simulink model "battery_charging_new"  (R2023a)
settings: Solver=ode23tb  StartTime=0.0  StopTime=350  RelTol=1e-3
undefined symbols (not defined in the file): Ion, Lithium
libraries: spsSeriesRLCBranchLib x3, spsCurrentMeasurementLib x2, spsDiodeLib x2, spsVoltageMeasurementLib x2, spsBatteryLib x1, spsMosfetLib x1, spsPVArrayLib x1, spsPWMGeneratorDCDCLib x1, spspowerguiLib x1
settings Model: Creator=mluser  LastModifiedBy=mluser
settings SolverCC: ZeroCrossAlgorithm=Adaptive
settings DebuggingCC: IgnoredZcDiagnostic=none

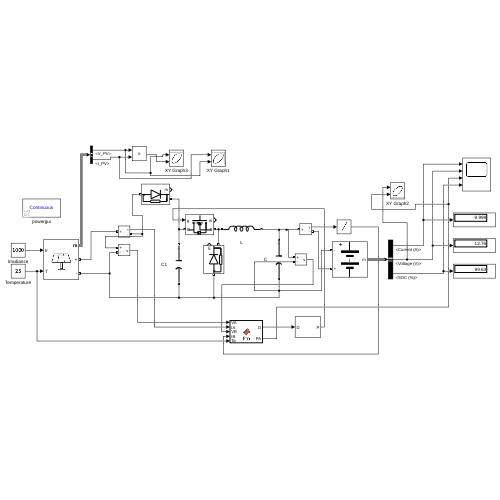
[thumbnail: Simulink's stored preview of the top-level diagram]
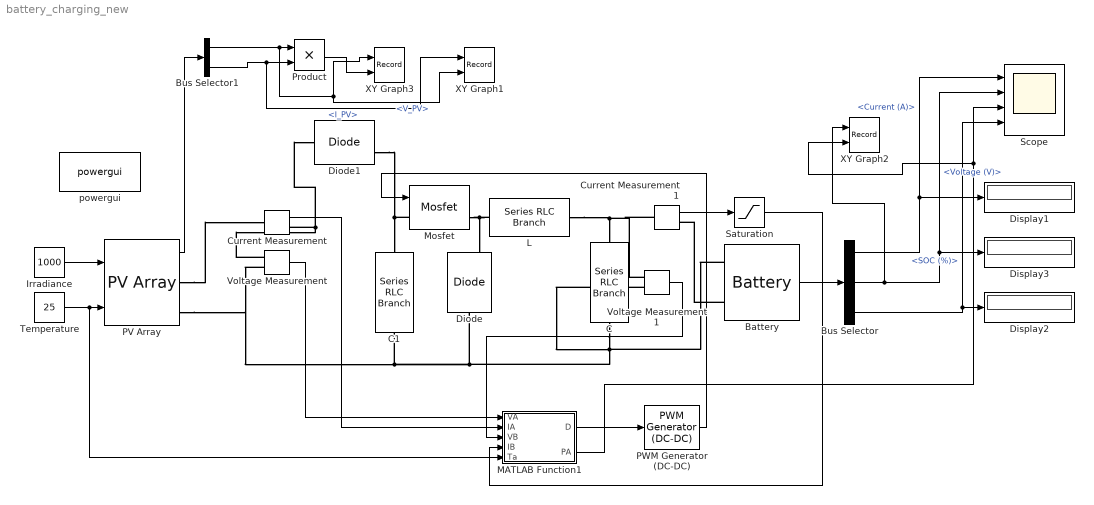
== system battery_charging_new ==
  Battery : spsBatteryLib/Battery  BatType=Lithium-Ion  ShowTempParam=off  ThermalPreset=no  ShowAgeParam=off  NomV=12  NomQ=50  SOC=99.6  Batt_Tr=30  PresetModel=off  MaxQ=50  MinV=9  FullV=14.4  Dis_rate=10  R=0.024  Normal_OP=25  expZone="[12.2171    0.166667]"  current=[6.5 13 32.5]  Units=Time  Tci=20  NomT=20  T2=-30  MaxQ2=4.8  FullV2=7.1  Normal_OP2=5.655  expZone2="[6.58           1]"  Rca=0.6  ti=2000  Dp=0  Neq0=0  Tsim=1e6  Ta1=25  Qeol=5.4*0.9  Reol=0.013333*1.2  Char_age=[2.3478, 3]  Dis_age=[2.3478, 10]  N1=1500  N2=10500  N3=1000  N4=1400  Ta2=45  N5=950
  Bus Selector : BusSelector  OutputSignals=Current (A),Voltage (V),SOC (%)
  Bus Selector1 : BusSelector  OutputSignals=V_PV,I_PV
  C : spsSeriesRLCBranchLib/Series RLC Branch  LConnTagsString=__new0  RConnTagsString=__new0  BranchType=C  Resistance=1  Inductance=1e-3  SetiL0=off  InitialCurrent=0  Capacitance=1000e-6  Setx0=off  InitialVoltage=0  Measurements=None
  C1 : spsSeriesRLCBranchLib/Series RLC Branch  LConnTagsString=__new0  RConnTagsString=__new0  BranchType=C  Resistance=1  Inductance=1e-3  SetiL0=off  InitialCurrent=0  Capacitance=1000e-6  Setx0=off  InitialVoltage=0  Measurements=None
  Current Measurement : spsCurrentMeasurementLib/Current Measurement  PhasorSimulation=off  OutputType=Complex  PSBequivalent=0
  Current Measurement1 : spsCurrentMeasurementLib/Current Measurement  PhasorSimulation=off  OutputType=Complex  PSBequivalent=0
  Diode : spsDiodeLib/Diode  Ron=0.001  Lon=0  Vf=0.8  IC=0  UseSnubber=0  Rs=500  Cs=250e-9  Measurements=on
  Diode1 : spsDiodeLib/Diode  Ron=0.001  Lon=0  Vf=0.8  IC=0  UseSnubber=0  Rs=500  Cs=250e-9  Measurements=on
  Display1 : Display
  Display2 : Display
  Display3 : Display
  Irradiance : Constant  Value=1000
  L : spsSeriesRLCBranchLib/Series RLC Branch  LConnTagsString=__new0  RConnTagsString=__new0  BranchType=L  Resistance=1  Inductance=10e-3  SetiL0=off  InitialCurrent=0  Capacitance=1e-6  Setx0=off  InitialVoltage=0  Measurements=None
  MATLAB Function1 : MATLAB Function  TreatAsAtomicUnit=on
  Mosfet : spsMosfetLib/Mosfet  Ron=0.1  Lon=0  Rd=0.01  Vfd=0  IC=0  Rs=1e5  Cs=inf  Measurements=on
  PV Array : spsPVArrayLib/PV Array  Npar=1  Nser=1  PlotType=array @ 1000 W/m2 & specified temperatures  S_vec="[ 1000  500  100 ]"  Temp_C_vec="[ 45 25  ]"  ModuleName=Canadian Solar Inc. CS6P-240MX  PlotWhenSelected=off  Pm=240.09  Ncell=60  Voc=37.3  Isc=8.46  Vm=30.2  Im=7.95  beta_Voc_pc=-0.35  alpha_Isc_pc=0.04  beta_Voc=-0.13055  alpha_Isc=0.003384  IL=8.4716  I0=1.9544e-10  nI=0.98841  Rsh=369.5316  Rs=0.32617  RobustModel=off  RobustCellTemperature=313.3991  BAL=on  Tc=1e-6  Tfilter=5e-5
  PWM Generator (DC-DC) : spsPWMGeneratorDCDCLib/PWM Generator (DC-DC)  Fsw=40000  Ts=0
  Product : Product
  Saturation : Saturate  UpperLimit=50  LowerLimit=0
  Scope : Scope  NumInputPorts=4
  Temperature : Constant  Value=25
  Voltage Measurement : spsVoltageMeasurementLib/Voltage Measurement  PhasorSimulation=off  OutputType=Complex  PSBequivalent=0
  Voltage Measurement1 : spsVoltageMeasurementLib/Voltage Measurement  PhasorSimulation=off  OutputType=Complex  PSBequivalent=0
  XY Graph1 : Record  FileSettingsInternal="{\"entries\":[{\"content\":{\"excelSettings\":{\"content\":{},\"type\":\"Streamout.ExcelSettings\"}},\"type\":\"Streamout.FileSettingStorage\",\"uuid\":\"\"}],\"packageUris\":[\"http:\\/\\/schema.mathworks.com\\/mf0\\/streamout_blocks\\/R2020a\"],\"version\":\"1.0\"}"  Layout=[1 1]  SignalsInternal="{\"entries\":[{\"content\":{\"signals\":[{\"content\":{\"blockPath\":[],\"dimensions\":[1],\"domain\":\"\",\"lineColor\":\"#a2142f\",\"plots\":[1],\"port\":1,\"sid\":[\"\"],\"signalID\":1211,\"signalName\":\"<I_PV>\"},\"type\":\"RecordBlkView.Signal\",\"uuid\":\"\"},{\"content\":{\"blockPath\":[],\"dimensions\":[1],\"domain\":\"\",\"lineColor\":\"#139fff\",\"plots\":[1],\"port\":2,\"sid\":[\"\"],\"signalID\":1215,\"signalName\":\"<V_PV>\"},\"type\":\"RecordBlkView.Signal\",\"uuid\":\"\"}]},\"type\":\"RecordBlkView.InputSignals\",\"uuid\":\"\"}],\"packageUris\":[\"http:\\/\\/schema.mathworks.com\\/mf0\\/streamout_blocks\\/R2020a\"],\"version\":\"1.0\"}"  VisualizationBindings="{\"xyplotplugin\":{\"info\":[{\"series\":[{\"bindingParametersList\":[{\"parameter\":\"X-Axis\",\"signalID\":1211,\"signalName\":\"<I_PV>\"},{\"parameter\":\"Y-Axis\",\"signalID\":1215,\"signalName\":\"<V_PV>\"}],\"seriesID\":56904}],\"subplotID\":1}]}}"  CompatibilityTag=XY  st=-1
  XY Graph2 : Record  FileSettingsInternal="{\"entries\":[{\"content\":{\"excelSettings\":{\"content\":{},\"type\":\"Streamout.ExcelSettings\"}},\"type\":\"Streamout.FileSettingStorage\",\"uuid\":\"\"}],\"packageUris\":[\"http:\\/\\/schema.mathworks.com\\/mf0\\/streamout_blocks\\/R2020a\"],\"version\":\"1.0\"}"  Layout=[1 1]  SignalsInternal="{\"entries\":[{\"content\":{\"signals\":[{\"content\":{\"blockPath\":[],\"dimensions\":[1],\"domain\":\"\",\"lineColor\":\"#a2142f\",\"plots\":[1],\"port\":1,\"sid\":[\"\"],\"signalID\":1219,\"signalName\":\"<Voltage (V)>\"},\"type\":\"RecordBlkView.Signal\",\"uuid\":\"\"},{\"content\":{\"blockPath\":[],\"dimensions\":[1],\"domain\":\"\",\"lineColor\":\"#139fff\",\"plots\":[1],\"port\":2,\"sid\":[\"\"],\"signalID\":1223,\"signalName\":\"MATLAB Function1:2\"},\"type\":\"RecordBlkView.Signal\",\"uuid\":\"\"}]},\"type\":\"RecordBlkView.InputSignals\",\"uuid\":\"\"}],\"packageUris\":[\"http:\\/\\/schema.mathworks.com\\/mf0\\/streamout_blocks\\/R2020a\"],\"version\":\"1.0\"}"  VisualizationBindings="{\"xyplotplugin\":{\"info\":[{\"series\":[{\"bindingParametersList\":[{\"parameter\":\"X-Axis\",\"signalID\":1219,\"signalName\":\"<Voltage (V)>\"},{\"parameter\":\"Y-Axis\",\"signalID\":1223,\"signalName\":\"MATLAB Function1:2\"}],\"seriesID\":36722}],\"subplotID\":1}]}}"  CompatibilityTag=XY  st=-1
  XY Graph3 : Record  FileSettingsInternal="{\"entries\":[{\"content\":{\"excelSettings\":{\"content\":{},\"type\":\"Streamout.ExcelSettings\"}},\"type\":\"Streamout.FileSettingStorage\",\"uuid\":\"\"}],\"packageUris\":[\"http:\\/\\/schema.mathworks.com\\/mf0\\/streamout_blocks\\/R2020a\"],\"version\":\"1.0\"}"  Layout=[1 1]  SignalsInternal="{\"entries\":[{\"content\":{\"signals\":[{\"content\":{\"blockPath\":[],\"dimensions\":[1],\"domain\":\"\",\"lineColor\":\"#a2142f\",\"plots\":[1],\"port\":1,\"sid\":[\"\"],\"signalID\":1227,\"signalName\":\"<V_PV>\"},\"type\":\"RecordBlkView.Signal\",\"uuid\":\"\"},{\"content\":{\"blockPath\":[],\"dimensions\":[1],\"domain\":\"\",\"lineColor\":\"#139fff\",\"plots\":[1],\"port\":2,\"sid\":[\"\"],\"signalID\":1231,\"signalName\":\"Product\"},\"type\":\"RecordBlkView.Signal\",\"uuid\":\"\"}]},\"type\":\"RecordBlkView.InputSignals\",\"uuid\":\"\"}],\"packageUris\":[\"http:\\/\\/schema.mathworks.com\\/mf0\\/streamout_blocks\\/R2020a\"],\"version\":\"1.0\"}"  VisualizationBindings="{\"xyplotplugin\":{\"info\":[{\"series\":[{\"bindingParametersList\":[{\"parameter\":\"X-Axis\",\"signalID\":1227,\"signalName\":\"<V_PV>\"},{\"parameter\":\"Y-Axis\",\"signalID\":1231,\"signalName\":\"Product\"}],\"seriesID\":53361}],\"subplotID\":1}]}}"  CompatibilityTag=XY  st=-1
  powergui : spspowerguiLib/powergui  Priority=1  SimulationMode=Continuous  SampleTime=1e-6  frequency=60  Iterations=50  frequencyindice=0  Pbase=100e6  ErrMax=1e-4  UnitsV=kV  UnitsW=MW  buscounter=0  FunctionMessages=off  echomessages=off  EnableUseOfTLC=off  CurrentSourceSwitches=off  DisableSnubberDevices=off  DisableRonSwitches=off  DisableVfSwitches=off  DisplayEquations=off  AutomaticDiscreteSolvers=off  SolverType=Tustin/Backward Euler (TBE)  Interpol=off  ExternalGateDelay=off  methode=off  Ts=100  x0status=blocks  SPID=on  SwTol=0  HookPort=off  NonlinearTolerance=1e-4  nMaxIteration=100  ContinueOnMaxIteration=off  RestoreLinks=warning  ResistiveCurrentMeasurement=off  Frange=[0:2:500]  Ylog=off  Xlog=on  ShowGrid=off  save=off  variable=ZData  structure=0  ZoomFFT=off  StartTime=0.0  cycles=1  DisplayStyle=1  fundamental=60  FreqAxis=off  MaxFrequency=1000  frequencyindicesteady=1  RmsSteady=1  display=off
  wires:
  Battery/1 -> Bus Selector/1
  Bus Selector/2 -> XY Graph2/1, Scope/2, Display3/1  "<Voltage (V)>"
  Bus Selector/3 -> Display2/1, Scope/4  "<SOC (%)>"
  Temperature/1 -> MATLAB Function1/5(Ta), PV Array/2
  Irradiance/1 -> PV Array/1
  Bus Selector/1 -> Scope/1, Display1/1  "<Current (A)>"
  Current Measurement/1 -> MATLAB Function1/2(IA)
  Voltage Measurement1/1 -> MATLAB Function1/3(VB)
  Voltage Measurement/1 -> MATLAB Function1/1(VA)
  MATLAB Function1/1(D) -> PWM Generator (DC-DC)/1
  PWM Generator (DC-DC)/1 -> Mosfet/1
  MATLAB Function1/2(PA) -> XY Graph2/2, Scope/3
  Current Measurement1/1 -> Saturation/1
  Saturation/1 -> MATLAB Function1/4(IB)
  PV Array/1 -> Bus Selector1/1
  Bus Selector1/1 -> XY Graph1/2, XY Graph3/1, Product/1  "<V_PV>"
  Bus Selector1/2 -> XY Graph1/1, Product/2  "<I_PV>"
  Product/1 -> XY Graph3/2
  connections:
  Mosfet/RConn1 -- L/LConn1 -- Diode/RConn1
  Battery/LConn2 -- Voltage Measurement1/LConn2 -- Voltage Measurement/LConn2 -- PV Array/RConn2 -- C1/RConn1 -- Diode/LConn1 -- C/RConn1
  L/RConn1 -- Current Measurement1/LConn1 -- Voltage Measurement1/LConn1 -- C/LConn1
  Voltage Measurement/LConn1 -- Current Measurement/RConn1 -- Diode1/LConn1
  PV Array/RConn1 -- Current Measurement/LConn1
  Battery/LConn1 -- Current Measurement1/RConn1
  Mosfet/LConn1 -- Diode1/RConn1 -- C1/LConn1

== matlab function battery_charging_new/MATLAB Function1 ==
  settings: updateMethod=DISCRETE
  data: VA input; IA input; VB input; IB input; D output; Ta input; PA output
function [D,PA]= fcn(VA, IA, VB, IB, Ta)
Nc=6;
alpha=-0.0035;
VBmin= 12.7+((Ta-25)*Nc*alpha);
VBmax= 14.4+((Ta-25)*Nc*alpha);
C=50;
IBmin=C/100;
ITrickle=0.2;
Beta=0.9;
DD=1e-6;

persistent   PAP VAP DP UP IBmax ;
if isempty(PAP)
  PAP=0;
  VAP=0;
  DP=0;
  UP=1;
  IBmax=C/5;
end

PA= VA*IA;
DPA=PA-PAP;
DVA=VA-VAP;
D=DP;

if IB>IBmax 
    UP=0;
elseif VB>VBmax && IB<IBmax
    if IBmax>IBmin
        IBmax=Beta*IBmax;
    else 
        IBmax=ITrickle;
    end 
else 
    if VB<VBmax && IB<IBmax
        UP=1;
    end 
    if VB<VBmin 
        IBmax=C/5;
    end 
end 

if UP==0 
    D=DP-DD;
elseif UP==1 
    if DPA>0
        if DVA>0
            D=DP-DD;
        elseif DVA<0
            D=DP+DD;
        end 
    elseif DPA<0
        if DVA>0
            D=DP+DD;
        elseif DVA<0
            D=DP-DD;
        end 
    end 
end 

if D>1
    D=1;
elseif D<0
    D=0;
end 

DP=D;
PAP=PA;
VAP=VA;
